simulink model "simulacion1"  (R2015a)
settings: Solver=ode3  StartTime=0.0  StopTime=10.0  FixedStep=1e-3  RelTol=1e-3
settings Model: Creator=Jesus  LastModifiedBy=Jesus

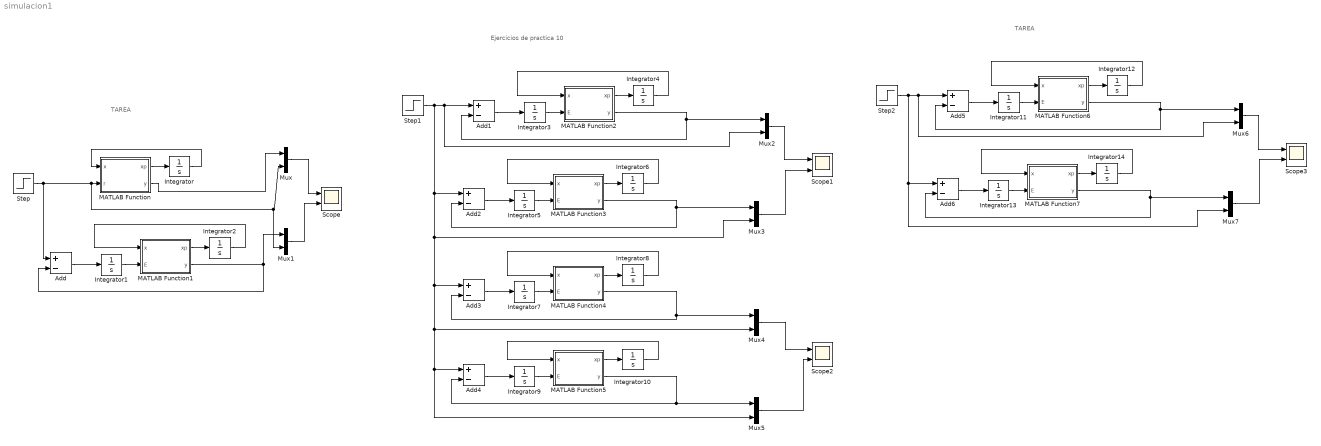
== system simulacion1 ==
  note: Ejercicios de practica 10
  note: TAREA
  note: TAREA
  Add{,1..6} (7 alike) : Sum  Inputs=+-
  Integrator : Integrator  InitialCondition=[0 0 0]
  Integrator{1,3,5,7,9,11,13} (7 alike) : Integrator
  Integrator10 : Integrator  InitialCondition=[0 0 0 0]
  Integrator12 : Integrator  InitialCondition=[0 0]
  Integrator14 : Integrator  InitialCondition=[0 0]
  Integrator2 : Integrator  InitialCondition=[0 0 0]
  Integrator4 : Integrator  InitialCondition=[0 0 0 0 0 0]
  Integrator6 : Integrator  InitialCondition=[0 0 0 0 0]
  Integrator8 : Integrator  InitialCondition=[0 0 0]
  MATLAB Function : MATLAB Function  TreatAsAtomicUnit=on
  MATLAB Function1 : MATLAB Function  TreatAsAtomicUnit=on
  MATLAB Function2 : MATLAB Function  TreatAsAtomicUnit=on
  MATLAB Function3 : MATLAB Function  TreatAsAtomicUnit=on
  MATLAB Function4 : MATLAB Function  TreatAsAtomicUnit=on
  MATLAB Function5 : MATLAB Function  TreatAsAtomicUnit=on
  MATLAB Function6 : MATLAB Function  TreatAsAtomicUnit=on
  MATLAB Function7 : MATLAB Function  TreatAsAtomicUnit=on
  Mux{,1..7} (8 alike) : Mux  Inputs=2
  Scope{,1..3} (4 alike) : Scope  NumInputPorts=2
      Scope settings: YMin=-5~-5  YMax=5~5
      Scope1 settings: YMin=-5~-5  YMax=5~5
      Scope2 settings: YMin=-5~-5  YMax=5~5  SaveName=ScopeData2
      Scope3 settings: YMin=-5~-5  YMax=5~5  SaveName=ScopeData3
  Step : Step  SampleTime=0
  Step1 : Step  SampleTime=0
  Step2 : Step  SampleTime=0
  wires:
  MATLAB Function/1(xp) -> Integrator/1
  Integrator/1 -> MATLAB Function/1(x)
  MATLAB Function/2(y) -> Mux/1
  Step/1 -> Add/1, Mux1/2, Mux/2, MATLAB Function/2(r)
  Mux/1 -> Scope/1
  MATLAB Function1/2(y) -> Add/2, Mux1/1
  Add/1 -> Integrator1/1
  Integrator1/1 -> MATLAB Function1/2(E)
  MATLAB Function1/1(xp) -> Integrator2/1
  Integrator2/1 -> MATLAB Function1/1(x)
  Mux1/1 -> Scope/2
  Add1/1 -> Integrator3/1
  Integrator3/1 -> MATLAB Function2/2(E)
  MATLAB Function2/1(xp) -> Integrator4/1
  Integrator4/1 -> MATLAB Function2/1(x)
  MATLAB Function2/2(y) -> Mux2/1, Add1/2
  Mux2/1 -> Scope1/1
  Add2/1 -> Integrator5/1
  Integrator5/1 -> MATLAB Function3/2(E)
  MATLAB Function3/1(xp) -> Integrator6/1
  Integrator6/1 -> MATLAB Function3/1(x)
  MATLAB Function3/2(y) -> Add2/2, Mux3/1
  Mux3/1 -> Scope1/2
  Add3/1 -> Integrator7/1
  Integrator7/1 -> MATLAB Function4/2(E)
  MATLAB Function4/1(xp) -> Integrator8/1
  Integrator8/1 -> MATLAB Function4/1(x)
  MATLAB Function4/2(y) -> Add3/2, Mux4/1
  Mux4/1 -> Scope2/1
  Add4/1 -> Integrator9/1
  Integrator9/1 -> MATLAB Function5/2(E)
  MATLAB Function5/1(xp) -> Integrator10/1
  Integrator10/1 -> MATLAB Function5/1(x)
  Step1/1 -> Add2/1, Add4/1, Mux5/2, Mux4/2, Add3/1, Mux3/2, Mux2/2, Add1/1
  MATLAB Function5/2(y) -> Mux5/1, Add4/2
  Mux5/1 -> Scope2/2
  Add5/1 -> Integrator11/1
  Integrator11/1 -> MATLAB Function6/2(E)
  MATLAB Function6/1(xp) -> Integrator12/1
  Integrator12/1 -> MATLAB Function6/1(x)
  MATLAB Function6/2(y) -> Add5/2, Mux6/1
  Mux6/1 -> Scope3/1
  Add6/1 -> Integrator13/1
  Integrator13/1 -> MATLAB Function7/2(E)
  MATLAB Function7/1(xp) -> Integrator14/1
  Integrator14/1 -> MATLAB Function7/1(x)
  MATLAB Function7/2(y) -> Mux7/1, Add6/2
  Mux7/1 -> Scope3/2
  Step2/1 -> Add5/1, Mux6/2, Mux7/2, Add6/1

== matlab function simulacion1/MATLAB Function1 ==
  data: xp output; x input; y output; E input
function [xp,y] = fcn(x,E)
%#codegen
K=[73.3787,17.6351,.3649];
KI=285.7143;
u=E*KI-K*x;
A=[0 1 0;0 0 1;-1 -5 -6];
B=[0 1 1]';
C=[1 0 0];
xp=A*x+B*u;
y = C*x;

== matlab function simulacion1/MATLAB Function ==
  data: xp output; x input; y output; r input
function [xp,y] = fcn(x,r)
%#codegen
K=[200 55 8];
u=r*K(1)-K*x;
A=[0 1 0;0 0 1;0 -5 -6];
B=[0 0 1]';
C=[1 0 0];
xp=A*x+B*u;
y = C*x;

== matlab function simulacion1/MATLAB Function2 ==
  data: xp output; x input; y output; E input
function [xp,y] = fcn(x,E)
%#codegen
K=[-0.5493 -0.1074 -0.3051 0.0024 1.4380 0.3843]*1e+4;
KI=7.8125e+03;
u=E*KI-K*x;
A=[0 1 0 0 0 0;-1 -1.5 1 .5 0 .5;0 0 0 1 0 0;2 1 -2 -2 0 1;0 0 0 0 0 1;0 1 0 1 0 -3];
B=[0 0 0 1 0 0]';
C=[0 0 0 0 1 0];
xp=A*x+B*u;
y = C*x;

== matlab function simulacion1/MATLAB Function3 ==
  data: xp output; x input; y output; E input
function [xp,y] = fcn(x,E)
%#codegen
K=[0.3784 0.0002 -0.2148 -0.4714 -1.2515]*1e+7;
KI=1638400;
u=E*KI-K*x;
A=[0 1 0 0 0;-9/50 0 3/5 0 0;0 0 0 1 0;3/10 0 -1 -1 0;0 3/10 0 0 0];
B=[0 1/50 0 0 0]';
C=[1 0 0 0 0];
xp=A*x+B*u;
y = C*x;

== matlab function simulacion1/MATLAB Function4 ==
  data: xp output; x input; y output; E input
function [xp,y] = fcn(x,E)
%#codegen
K=[-276.1000 468.1000 0];
KI=192.0000;
u=E*KI-K*x;
A=[-25/18 0 0;-5/6 0 0;-1/12 0 0];
B=[25/18 5/6 1/12]';
C=[0 0 1];
xp=A*x+B*u;
y = C*x;

== matlab function simulacion1/MATLAB Function5 ==
  data: xp output; x input; y output; E input
function [xp,y] = fcn(x,E)
%#codegen
K=[-0.7604 0.0770 4.1934 3.4330]*1e+3;
KI=3.5100e+03;
u=E*KI-K*x;
A=[0 1 0 0;-11/26 -40/13 0 0;0 1/10 0 0;0 1/5 0 0];
B=[0 1/13 0 0]';
C=[0 0 1 0];
xp=A*x+B*u;
y = C*x;

== matlab function simulacion1/MATLAB Function6 ==
  data: xp output; x input; y output; E input
function [xp,y] = fcn(x,E)
%#codegen
K=[820.0281 51.0000];
KI=7.3211e+03;
u=E*KI-K*x;
A=[0 1;-3 -5];
B=[0 1]';
C=[1 0];
xp=A*x+B*u;
y = C*x;

== matlab function simulacion1/MATLAB Function7 ==
  data: xp output; x input; y output; E input
function [xp,y] = fcn(x,E)
%#codegen
K=[5.1354 0.1310]*1.0e+03;
KI=1.1444e+05;
u=E*KI-K*x;
A=[0 1;-7 -9];
B=[0 1]';
C=[1 0];
xp=A*x+B*u;
y = C*x;
